simulink model "final_quadruped_180622_veldelay"  (R2021a)
settings: Solver=ode15s  StartTime=0.0  StopTime=2  FixedStep=1e-3  RelTol=1e-5  EnableMultiTasking=on
values from neighbouring files (symbols this model uses):
  foot_x = 8    [bipedparameters.m]    (also in fcn.m; finalrobotParameters.m; finalrobotParameters_110522.m; finalrobotParameters_140522.m)
  foot_y = 6    [bipedparameters.m]    (also in fcn.m; finalrobotParameters.m; finalrobotParameters_110522.m; finalrobotParameters_140522.m)
  foot_z = 1    [bipedparameters.m]    (also in fcn.m; finalrobotParameters.m; finalrobotParameters_110522.m; finalrobotParameters_140522.m)
  height_plane = 0.025    [bipedparameters.m]    (also in finalrobotParameters.m; finalrobotParameters_110522.m; finalrobotParameters_140522.m; finalrobotParameters_240522.m)
  kd_ankle = 1000    [bipedparameters.m]    (also in finalrobotParameters_240522.m)
  kd_hip = 1000    [bipedparameters.m]    (also in finalrobotParameters_240522.m)
  kd_knee = 1000    [bipedparameters.m]    (also in finalrobotParameters_240522.m)
  ki_ankle = 1000    [bipedparameters.m]    (also in finalrobotParameters_240522.m)
  ki_hip = 1000    [bipedparameters.m]    (also in finalrobotParameters_240522.m)
  ki_knee = 2000    [bipedparameters.m]    (also in finalrobotParameters_240522.m)
  kp_ankle = 1000    [bipedparameters.m]    (also in finalrobotParameters_240522.m)
  kp_hip = 1000    [bipedparameters.m]    (also in finalrobotParameters_240522.m)
  kp_knee = 2000    [bipedparameters.m]    (also in finalrobotParameters_240522.m)
  lower_leg_length = 10    [bipedparameters.m]    (also in fcn.m; finalrobotParameters.m; finalrobotParameters_110522.m; finalrobotParameters_140522.m)
  m_ll = density*leg_radius*leg_radius*lower_leg_length*3.141592653589*0.01*0.01*0.01    (= 0.0176714586764)    [bipedparameters.m]    (also in fcn.m; finalrobotParameters_140522.m; finalrobotParameters_240522.m; hdotlb.m)
  m_ul = density*leg_radius*leg_radius*upper_leg_length*3.141592653589*0.01*0.01*0.01    (= 0.0176714586764)    [bipedparameters.m]    (also in fcn.m; finalrobotParameters_140522.m; finalrobotParameters_240522.m; hdotlb.m)
  plane_x = 25    [bipedparameters.m]    (also in finalrobotParameters.m; finalrobotParameters_110522.m; finalrobotParameters_140522.m; finalrobotParameters_240522.m)
  plane_y = 3    [bipedparameters.m]    (also in finalrobotParameters.m; finalrobotParameters_110522.m; finalrobotParameters_140522.m; finalrobotParameters_240522.m)
  torso_offset_x = -0.5    [bipedparameters.m]    (also in finalrobotParameters.m = 10; finalrobotParameters_110522.m = 10; finalrobotParameters_140522.m = 10; finalrobotParameters_240522.m = 10)
  torso_offset_z = -2    [bipedparameters.m]    (also in finalrobotParameters.m; finalrobotParameters_110522.m; finalrobotParameters_140522.m; finalrobotParameters_240522.m)
  torso_x = 5    [bipedparameters.m]    (also in fcn.m = 25; finalrobotParameters.m = 25; finalrobotParameters_110522.m = 25; finalrobotParameters_140522.m = 25)
  torso_y = 10    [bipedparameters.m]    (also in fcn.m = 16; finalrobotParameters.m = 16; finalrobotParameters_110522.m = 16; finalrobotParameters_140522.m = 16)
  torso_z = 8    [bipedparameters.m]    (also in fcn.m = 10; finalrobotParameters.m = 10; finalrobotParameters_110522.m = 10; finalrobotParameters_140522.m = 10)
  upper_leg_length = 10    [bipedparameters.m]    (also in fcn.m; finalrobotParameters.m; finalrobotParameters_110522.m; finalrobotParameters_140522.m)
undefined symbols (not defined in the file or in its folder): sigbuilder_block, X, Y, Z
libraries: nesl_utility x188, sm_lib x71, Contact_Forces_Lib x16, pid_lib x12, fl_lib x3
(part 2 of 8)

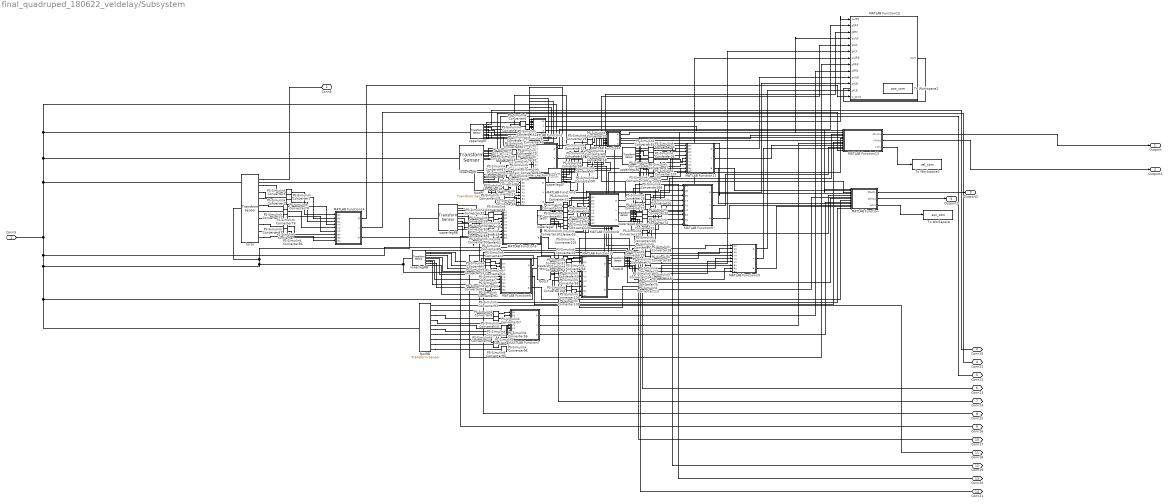
== system final_quadruped_180622_veldelay/Subsystem ==
  MATLAB Function : MATLAB Function  TreatAsAtomicUnit=on
  MATLAB Function1 : MATLAB Function  TreatAsAtomicUnit=on
  MATLAB Function10 : MATLAB Function  TreatAsAtomicUnit=on
  MATLAB Function11 : MATLAB Function  TreatAsAtomicUnit=on
  MATLAB Function12 : MATLAB Function  TreatAsAtomicUnit=on
  MATLAB Function13 : MATLAB Function  TreatAsAtomicUnit=on
  MATLAB Function14 : MATLAB Function  TreatAsAtomicUnit=on
  MATLAB Function15 : MATLAB Function  TreatAsAtomicUnit=on
  MATLAB Function2 : MATLAB Function  TreatAsAtomicUnit=on
  MATLAB Function3 : MATLAB Function  TreatAsAtomicUnit=on
  MATLAB Function4 : MATLAB Function  TreatAsAtomicUnit=on
  MATLAB Function5 : MATLAB Function  TreatAsAtomicUnit=on
  MATLAB Function6 : MATLAB Function  TreatAsAtomicUnit=on
  MATLAB Function7 : MATLAB Function  TreatAsAtomicUnit=on
  MATLAB Function8 : MATLAB Function  TreatAsAtomicUnit=on
  MATLAB Function9 : MATLAB Function  TreatAsAtomicUnit=on
  PS-Simulink Converter{,1..114} (115 alike) : nesl_utility/PS-Simulink Converter  PhysicalDomain=network_engine_domain  SubClassName=ps_output  LeftPortType=input  RightPortType=output  PseudoPeriodic=off  Frequencies=[]  Unit=inherit  AffineConversion=off
      settings: SourceProductBaseCode=PW,SS
  To Workspace : ToWorkspace  VariableName=acc_com  SaveFormat=Timeseries  SampleTime=-1
  To Workspace1 : ToWorkspace  VariableName=vel_com  SaveFormat=Timeseries  SampleTime=-1
  To Workspace2 : ToWorkspace  VariableName=pos_com  SaveFormat=Timeseries  SampleTime=-1
  footLB : sm_lib/Frames and Transforms/Transform Sensor  MeasurementFrame=World  SenseAngle=off  SenseAxis=off  SenseAngle1=off  SenseAngle2=off  SenseAngle3=off  SenseQ=off  SenseR=off  SenseOmegaX=off  SenseOmegaY=off  SenseOmegaZ=off  SenseOmega1=off  SenseOmega2=off  SenseOmega3=off  SenseQDot=off  SenseRDot=off  SenseAlphaX=off  SenseAlphaY=off  SenseAlphaZ=off  SenseAlpha1=off  SenseAlpha2=off  SenseAlpha3=off  SenseQDDot=off  SenseRDDot=off  SenseX=on  SenseY=on  SenseZ=on  SenseRad=off  SenseAzim=off  SenseDist=off  SenseInc=off  SenseXDot=on  SenseYDot=on  SenseZDot=on  SenseRadDot=off  SenseAzimDot=off  SenseDistDot=off  SenseIncDot=off  SenseXDDot=on  SenseYDDot=on  SenseZDDot=on  SenseRadDDot=off  SenseAzimDDot=off  SenseDistDDot=off  SenseIncDDot=off
  footLF : sm_lib/Frames and Transforms/Transform Sensor  MeasurementFrame=World  SenseAngle=off  SenseAxis=off  SenseAngle1=off  SenseAngle2=off  SenseAngle3=off  SenseQ=off  SenseR=off  SenseOmegaX=off  SenseOmegaY=off  SenseOmegaZ=off  SenseOmega1=off  SenseOmega2=off  SenseOmega3=off  SenseQDot=off  SenseRDot=off  SenseAlphaX=off  SenseAlphaY=off  SenseAlphaZ=off  SenseAlpha1=off  SenseAlpha2=off  SenseAlpha3=off  SenseQDDot=off  SenseRDDot=off  SenseX=on  SenseY=on  SenseZ=on  SenseRad=off  SenseAzim=off  SenseDist=off  SenseInc=off  SenseXDot=on  SenseYDot=on  SenseZDot=on  SenseRadDot=off  SenseAzimDot=off  SenseDistDot=off  SenseIncDot=off  SenseXDDot=on  SenseYDDot=on  SenseZDDot=on  SenseRadDDot=off  SenseAzimDDot=off  SenseDistDDot=off  SenseIncDDot=off
  footRB : sm_lib/Frames and Transforms/Transform Sensor  MeasurementFrame=World  SenseAngle=off  SenseAxis=off  SenseAngle1=off  SenseAngle2=off  SenseAngle3=off  SenseQ=off  SenseR=off  SenseOmegaX=off  SenseOmegaY=off  SenseOmegaZ=off  SenseOmega1=off  SenseOmega2=off  SenseOmega3=off  SenseQDot=off  SenseRDot=off  SenseAlphaX=off  SenseAlphaY=off  SenseAlphaZ=off  SenseAlpha1=off  SenseAlpha2=off  SenseAlpha3=off  SenseQDDot=off  SenseRDDot=off  SenseX=on  SenseY=on  SenseZ=on  SenseRad=off  SenseAzim=off  SenseDist=off  SenseInc=off  SenseXDot=on  SenseYDot=on  SenseZDot=on  SenseRadDot=off  SenseAzimDot=off  SenseDistDot=off  SenseIncDot=off  SenseXDDot=on  SenseYDDot=on  SenseZDDot=on  SenseRadDDot=off  SenseAzimDDot=off  SenseDistDDot=off  SenseIncDDot=off
  footRF : sm_lib/Frames and Transforms/Transform Sensor  MeasurementFrame=World  SenseAngle=off  SenseAxis=off  SenseAngle1=off  SenseAngle2=off  SenseAngle3=off  SenseQ=off  SenseR=off  SenseOmegaX=off  SenseOmegaY=off  SenseOmegaZ=off  SenseOmega1=off  SenseOmega2=off  SenseOmega3=off  SenseQDot=off  SenseRDot=off  SenseAlphaX=off  SenseAlphaY=off  SenseAlphaZ=off  SenseAlpha1=off  SenseAlpha2=off  SenseAlpha3=off  SenseQDDot=off  SenseRDDot=off  SenseX=on  SenseY=on  SenseZ=on  SenseRad=off  SenseAzim=off  SenseDist=off  SenseInc=off  SenseXDot=on  SenseYDot=on  SenseZDot=on  SenseRadDot=off  SenseAzimDot=off  SenseDistDot=off  SenseIncDot=off  SenseXDDot=on  SenseYDDot=on  SenseZDDot=on  SenseRadDDot=off  SenseAzimDDot=off  SenseDistDDot=off  SenseIncDDot=off
  lowerlegLB : sm_lib/Frames and Transforms/Transform Sensor  MeasurementFrame=World  SenseAngle=off  SenseAxis=off  SenseAngle1=off  SenseAngle2=off  SenseAngle3=off  SenseQ=off  SenseR=off  SenseOmegaX=off  SenseOmegaY=off  SenseOmegaZ=off  SenseOmega1=off  SenseOmega2=off  SenseOmega3=off  SenseQDot=off  SenseRDot=off  SenseAlphaX=off  SenseAlphaY=off  SenseAlphaZ=off  SenseAlpha1=off  SenseAlpha2=off  SenseAlpha3=off  SenseQDDot=off  SenseRDDot=off  SenseX=on  SenseY=on  SenseZ=on  SenseRad=off  SenseAzim=off  SenseDist=off  SenseInc=off  SenseXDot=on  SenseYDot=on  SenseZDot=on  SenseRadDot=off  SenseAzimDot=off  SenseDistDot=off  SenseIncDot=off  SenseXDDot=on  SenseYDDot=on  SenseZDDot=on  SenseRadDDot=off  SenseAzimDDot=off  SenseDistDDot=off  SenseIncDDot=off
  lowerlegLF : sm_lib/Frames and Transforms/Transform Sensor  MeasurementFrame=World  SenseAngle=off  SenseAxis=off  SenseAngle1=off  SenseAngle2=off  SenseAngle3=off  SenseQ=off  SenseR=off  SenseOmegaX=off  SenseOmegaY=off  SenseOmegaZ=off  SenseOmega1=off  SenseOmega2=off  SenseOmega3=off  SenseQDot=off  SenseRDot=off  SenseAlphaX=off  SenseAlphaY=off  SenseAlphaZ=off  SenseAlpha1=off  SenseAlpha2=off  SenseAlpha3=off  SenseQDDot=off  SenseRDDot=off  SenseX=on  SenseY=on  SenseZ=on  SenseRad=off  SenseAzim=off  SenseDist=off  SenseInc=off  SenseXDot=on  SenseYDot=on  SenseZDot=on  SenseRadDot=off  SenseAzimDot=off  SenseDistDot=off  SenseIncDot=off  SenseXDDot=on  SenseYDDot=on  SenseZDDot=on  SenseRadDDot=off  SenseAzimDDot=off  SenseDistDDot=off  SenseIncDDot=off
  lowerlegRB : sm_lib/Frames and Transforms/Transform Sensor  MeasurementFrame=World  SenseAngle=off  SenseAxis=off  SenseAngle1=off  SenseAngle2=off  SenseAngle3=off  SenseQ=off  SenseR=off  SenseOmegaX=off  SenseOmegaY=off  SenseOmegaZ=off  SenseOmega1=off  SenseOmega2=off  SenseOmega3=off  SenseQDot=off  SenseRDot=off  SenseAlphaX=off  SenseAlphaY=off  SenseAlphaZ=off  SenseAlpha1=off  SenseAlpha2=off  SenseAlpha3=off  SenseQDDot=off  SenseRDDot=off  SenseX=on  SenseY=on  SenseZ=on  SenseRad=off  SenseAzim=off  SenseDist=off  SenseInc=off  SenseXDot=on  SenseYDot=on  SenseZDot=on  SenseRadDot=off  SenseAzimDot=off  SenseDistDot=off  SenseIncDot=off  SenseXDDot=on  SenseYDDot=on  SenseZDDot=on  SenseRadDDot=off  SenseAzimDDot=off  SenseDistDDot=off  SenseIncDDot=off
  lowerlegRF : sm_lib/Frames and Transforms/Transform Sensor  MeasurementFrame=World  SenseAngle=off  SenseAxis=off  SenseAngle1=off  SenseAngle2=off  SenseAngle3=off  SenseQ=off  SenseR=off  SenseOmegaX=off  SenseOmegaY=off  SenseOmegaZ=off  SenseOmega1=off  SenseOmega2=off  SenseOmega3=off  SenseQDot=off  SenseRDot=off  SenseAlphaX=off  SenseAlphaY=off  SenseAlphaZ=off  SenseAlpha1=off  SenseAlpha2=off  SenseAlpha3=off  SenseQDDot=off  SenseRDDot=off  SenseX=on  SenseY=on  SenseZ=on  SenseRad=off  SenseAzim=off  SenseDist=off  SenseInc=off  SenseXDot=on  SenseYDot=on  SenseZDot=on  SenseRadDot=off  SenseAzimDot=off  SenseDistDot=off  SenseIncDot=off  SenseXDDot=on  SenseYDDot=on  SenseZDDot=on  SenseRadDDot=off  SenseAzimDDot=off  SenseDistDDot=off  SenseIncDDot=off
  torso : sm_lib/Frames and Transforms/Transform Sensor  MeasurementFrame=World  SenseAngle=off  SenseAxis=off  SenseAngle1=off  SenseAngle2=off  SenseAngle3=off  SenseQ=off  SenseR=off  SenseOmegaX=off  SenseOmegaY=off  SenseOmegaZ=off  SenseOmega1=off  SenseOmega2=off  SenseOmega3=off  SenseQDot=off  SenseRDot=off  SenseAlphaX=off  SenseAlphaY=off  SenseAlphaZ=off  SenseAlpha1=off  SenseAlpha2=off  SenseAlpha3=off  SenseQDDot=off  SenseRDDot=off  SenseX=on  SenseY=on  SenseZ=on  SenseRad=off  SenseAzim=off  SenseDist=off  SenseInc=off  SenseXDot=on  SenseYDot=on  SenseZDot=on  SenseRadDot=off  SenseAzimDot=off  SenseDistDot=off  SenseIncDot=off  SenseXDDot=on  SenseYDDot=on  SenseZDDot=on  SenseRadDDot=off  SenseAzimDDot=off  SenseDistDDot=off  SenseIncDDot=off
  upperlegLB1 : sm_lib/Frames and Transforms/Transform Sensor  MeasurementFrame=World  SenseAngle=off  SenseAxis=off  SenseAngle1=off  SenseAngle2=off  SenseAngle3=off  SenseQ=off  SenseR=off  SenseOmegaX=off  SenseOmegaY=off  SenseOmegaZ=off  SenseOmega1=off  SenseOmega2=off  SenseOmega3=off  SenseQDot=off  SenseRDot=off  SenseAlphaX=off  SenseAlphaY=off  SenseAlphaZ=off  SenseAlpha1=off  SenseAlpha2=off  SenseAlpha3=off  SenseQDDot=off  SenseRDDot=off  SenseX=on  SenseY=on  SenseZ=on  SenseRad=off  SenseAzim=off  SenseDist=off  SenseInc=off  SenseXDot=on  SenseYDot=on  SenseZDot=on  SenseRadDot=off  SenseAzimDot=off  SenseDistDot=off  SenseIncDot=off  SenseXDDot=on  SenseYDDot=on  SenseZDDot=on  SenseRadDDot=off  SenseAzimDDot=off  SenseDistDDot=off  SenseIncDDot=off
  upperlegLF : sm_lib/Frames and Transforms/Transform Sensor  MeasurementFrame=World  SenseAngle=off  SenseAxis=off  SenseAngle1=off  SenseAngle2=off  SenseAngle3=off  SenseQ=off  SenseR=off  SenseOmegaX=off  SenseOmegaY=off  SenseOmegaZ=off  SenseOmega1=off  SenseOmega2=off  SenseOmega3=off  SenseQDot=off  SenseRDot=off  SenseAlphaX=off  SenseAlphaY=off  SenseAlphaZ=off  SenseAlpha1=off  SenseAlpha2=off  SenseAlpha3=off  SenseQDDot=off  SenseRDDot=off  SenseX=on  SenseY=on  SenseZ=on  SenseRad=off  SenseAzim=off  SenseDist=off  SenseInc=off  SenseXDot=on  SenseYDot=on  SenseZDot=on  SenseRadDot=off  SenseAzimDot=off  SenseDistDot=off  SenseIncDot=off  SenseXDDot=on  SenseYDDot=on  SenseZDDot=on  SenseRadDDot=off  SenseAzimDDot=off  SenseDistDDot=off  SenseIncDDot=off
  upperlegRB : sm_lib/Frames and Transforms/Transform Sensor  MeasurementFrame=World  SenseAngle=off  SenseAxis=off  SenseAngle1=off  SenseAngle2=off  SenseAngle3=off  SenseQ=off  SenseR=off  SenseOmegaX=off  SenseOmegaY=off  SenseOmegaZ=off  SenseOmega1=off  SenseOmega2=off  SenseOmega3=off  SenseQDot=off  SenseRDot=off  SenseAlphaX=off  SenseAlphaY=off  SenseAlphaZ=off  SenseAlpha1=off  SenseAlpha2=off  SenseAlpha3=off  SenseQDDot=off  SenseRDDot=off  SenseX=on  SenseY=on  SenseZ=on  SenseRad=off  SenseAzim=off  SenseDist=off  SenseInc=off  SenseXDot=on  SenseYDot=on  SenseZDot=on  SenseRadDot=off  SenseAzimDot=off  SenseDistDot=off  SenseIncDot=off  SenseXDDot=on  SenseYDDot=on  SenseZDDot=on  SenseRadDDot=off  SenseAzimDDot=off  SenseDistDDot=off  SenseIncDDot=off
  upperlegRF : sm_lib/Frames and Transforms/Transform Sensor  MeasurementFrame=World  SenseAngle=off  SenseAxis=off  SenseAngle1=off  SenseAngle2=off  SenseAngle3=off  SenseQ=off  SenseR=off  SenseOmegaX=off  SenseOmegaY=off  SenseOmegaZ=off  SenseOmega1=off  SenseOmega2=off  SenseOmega3=off  SenseQDot=off  SenseRDot=off  SenseAlphaX=off  SenseAlphaY=off  SenseAlphaZ=off  SenseAlpha1=off  SenseAlpha2=off  SenseAlpha3=off  SenseQDDot=off  SenseRDDot=off  SenseX=on  SenseY=on  SenseZ=on  SenseRad=off  SenseAzim=off  SenseDist=off  SenseInc=off  SenseXDot=on  SenseYDot=on  SenseZDot=on  SenseRadDot=off  SenseAzimDot=off  SenseDistDot=off  SenseIncDot=off  SenseXDDot=on  SenseYDDot=on  SenseZDDot=on  SenseRadDDot=off  SenseAzimDDot=off  SenseDistDDot=off  SenseIncDDot=off
  Conn5 : PMIOPort  Side=Left
  Conn4 : PMIOPort  Port=2  Side=Right
  Conn10 : PMIOPort  Port=3  Side=Right
  Conn11 : PMIOPort  Port=4  Side=Right
  Conn12 : PMIOPort  Port=5  Side=Right
  Conn13 : PMIOPort  Port=6  Side=Right
  Conn14 : PMIOPort  Port=7  Side=Right
  Conn15 : PMIOPort  Port=8  Side=Right
  Conn16 : PMIOPort  Port=9  Side=Right
  Conn17 : PMIOPort  Port=10  Side=Right
  Conn18 : PMIOPort  Port=11  Side=Right
  Conn19 : PMIOPort  Port=12  Side=Right
  Conn20 : PMIOPort  Port=13  Side=Right
  Conn21 : PMIOPort  Port=14  Side=Right
  Outport : Outport
  Outport1 : Outport  Port=2
  Outport2 : Outport  Port=3
  Outport3 : Outport  Port=4
  wires:
  PS-Simulink Converter10/1 -> MATLAB Function7/2(py)
  PS-Simulink Converter13/1 -> MATLAB Function2/1(px)
  MATLAB Function12/2(v) -> MATLAB Function13/10(vulLB)
  PS-Simulink Converter36/1 -> MATLAB Function12/3(pz)
  PS-Simulink Converter14/1 -> MATLAB Function2/2(py)
  PS-Simulink Converter9/1 -> MATLAB Function7/1(px)
  PS-Simulink Converter11/1 -> MATLAB Function7/3(pz)
  PS-Simulink Converter8/1 -> MATLAB Function1/2(py)
  PS-Simulink Converter7/1 -> MATLAB Function6/3(pz)
  PS-Simulink Converter38/1 -> MATLAB Function5/2(py)
  PS-Simulink Converter16/1 -> MATLAB Function3/4(vx)
  MATLAB Function9/2(v) -> MATLAB Function13/11(vllLB)
  MATLAB Function1/2(v) -> MATLAB Function13/1(vulRF)
  PS-Simulink Converter17/1 -> MATLAB Function3/5(vy)
  PS-Simulink Converter28/1 -> MATLAB Function10/1(px)
  PS-Simulink Converter21/1 -> MATLAB Function4/3(pz)
  PS-Simulink Converter18/1 -> MATLAB Function3/6(vz)
  PS-Simulink Converter6/1 -> MATLAB Function1/1(px)
  PS-Simulink Converter19/1 -> MATLAB Function4/1(px)
  PS-Simulink Converter5/1 -> MATLAB Function6/2(py)
  PS-Simulink Converter20/1 -> MATLAB Function4/2(py)
  PS-Simulink Converter12/1 -> MATLAB Function1/3(pz)
  PS-Simulink Converter15/1 -> MATLAB Function2/3(pz)
  PS-Simulink Converter39/1 -> MATLAB Function5/3(pz)
  MATLAB Function2/2(v) -> MATLAB Function13/2(vllRF)
  MATLAB Function10/2(v) -> MATLAB Function13/12(vfLB)
  PS-Simulink Converter27/1 -> MATLAB Function9/3(pz)
  PS-Simulink Converter4/1 -> MATLAB Function6/1(px)
  PS-Simulink Converter25/1 -> MATLAB Function9/1(px)
  PS-Simulink Converter37/1 -> MATLAB Function5/1(px)
  PS-Simulink Converter26/1 -> MATLAB Function9/2(py)
  PS-Simulink Converter24/1 -> MATLAB Function8/3(pz)
  PS-Simulink Converter22/1 -> MATLAB Function8/1(px)
  PS-Simulink Converter23/1 -> MATLAB Function8/2(py)
  PS-Simulink Converter34/1 -> MATLAB Function12/1(px)
  PS-Simulink Converter35/1 -> MATLAB Function12/2(py)
  MATLAB Function7/2(v) -> MATLAB Function13/9(vfRB)
  MATLAB Function6/2(v) -> MATLAB Function13/8(vllRB)
  MATLAB Function5/2(v) -> MATLAB Function13/7(vulRB)
  MATLAB Function11/2(v) -> MATLAB Function13/6(vfLF)
  PS-Simulink Converter33/1 -> MATLAB Function11/3(pz)
  MATLAB Function8/2(v) -> MATLAB Function13/5(vllLF)
  MATLAB Function4/2(v) -> MATLAB Function13/4(vulLF)
  MATLAB Function3/2(v) -> MATLAB Function13/3(vfRF)
  PS-Simulink Converter32/1 -> MATLAB Function11/2(py)
  PS-Simulink Converter31/1 -> MATLAB Function11/1(px)
  PS-Simulink Converter30/1 -> MATLAB Function10/3(pz)
  PS-Simulink Converter29/1 -> MATLAB Function10/2(py)
  PS-Simulink Converter3/1 -> MATLAB Function14/1(px)
  PS-Simulink Converter1/1 -> MATLAB Function14/2(py)
  PS-Simulink Converter2/1 -> MATLAB Function14/3(pz)
  MATLAB Function14/2(v) -> MATLAB Function13/13(v_torso)
  MATLAB Function13/1(Mvcm) -> Outport/1
  MATLAB Function13/2(vlinks) -> Outport1/1
  PS-Simulink Converter40/1 -> MATLAB Function1/4(vx)
  PS-Simulink Converter41/1 -> MATLAB Function1/5(vy)
  PS-Simulink Converter42/1 -> MATLAB Function1/6(vz)
  PS-Simulink Converter43/1 -> MATLAB Function2/4(vx)
  PS-Simulink Converter44/1 -> MATLAB Function2/5(vy)
  PS-Simulink Converter45/1 -> MATLAB Function2/6(vz)
  PS-Simulink Converter46/1 -> MATLAB Function3/7(ax)
  PS-Simulink Converter47/1 -> MATLAB Function3/8(ay)
  PS-Simulink Converter48/1 -> MATLAB Function3/9(az)
  PS-Simulink Converter49/1 -> MATLAB Function5/4(vx)
  PS-Simulink Converter50/1 -> MATLAB Function5/5(vy)
  PS-Simulink Converter51/1 -> MATLAB Function5/6(vz)
  PS-Simulink Converter52/1 -> MATLAB Function6/4(vx)
  PS-Simulink Converter53/1 -> MATLAB Function6/5(vy)
  PS-Simulink Converter54/1 -> MATLAB Function6/6(vz)
  PS-Simulink Converter55/1 -> MATLAB Function7/5(vy)
  PS-Simulink Converter57/1 -> MATLAB Function7/4(vx)
  PS-Simulink Converter56/1 -> MATLAB Function7/6(vz)
  PS-Simulink Converter58/1 -> MATLAB Function4/4(vx)
  PS-Simulink Converter59/1 -> MATLAB Function4/5(vy)
  PS-Simulink Converter60/1 -> MATLAB Function4/6(vz)
  PS-Simulink Converter61/1 -> MATLAB Function8/4(vx)
  PS-Simulink Converter62/1 -> MATLAB Function8/5(vy)
  PS-Simulink Converter63/1 -> MATLAB Function8/6(vz)
  PS-Simulink Converter64/1 -> MATLAB Function11/4(vx)
  PS-Simulink Converter65/1 -> MATLAB Function11/5(vy)
  PS-Simulink Converter66/1 -> MATLAB Function11/6(vz)
  PS-Simulink Converter67/1 -> MATLAB Function12/4(vx)
  PS-Simulink Converter68/1 -> MATLAB Function12/5(vy)
  PS-Simulink Converter69/1 -> MATLAB Function12/6(vz)
  PS-Simulink Converter70/1 -> MATLAB Function9/4(vx)
  PS-Simulink Converter71/1 -> MATLAB Function9/5(vy)
  PS-Simulink Converter72/1 -> MATLAB Function9/6(vz)
  PS-Simulink Converter73/1 -> MATLAB Function10/4(vx)
  PS-Simulink Converter74/1 -> MATLAB Function10/5(vy)
  PS-Simulink Converter75/1 -> MATLAB Function10/6(vz)
  PS-Simulink Converter78/1 -> MATLAB Function14/4(vx)
  PS-Simulink Converter76/1 -> MATLAB Function14/5(vy)
  PS-Simulink Converter77/1 -> MATLAB Function14/6(vz)
  MATLAB Function14/3(a) -> MATLAB Function/13(a_torso)
  MATLAB Function1/3(a) -> MATLAB Function/1(aulRF)
  MATLAB Function2/3(a) -> MATLAB Function/2(allRF)
  MATLAB Function3/3(a) -> MATLAB Function/3(afRF)
  MATLAB Function4/3(a) -> MATLAB Function/4(aulLF)
  MATLAB Function8/3(a) -> MATLAB Function/5(allLF)
  MATLAB Function11/3(a) -> MATLAB Function/6(afLF)
  MATLAB Function5/3(a) -> MATLAB Function/7(aulRB)
  MATLAB Function6/3(a) -> MATLAB Function/8(allRB)
  MATLAB Function7/3(a) -> MATLAB Function/9(afRB)
  MATLAB Function12/3(a) -> MATLAB Function/10(aulLB)
  MATLAB Function9/3(a) -> MATLAB Function/11(allLB)
  MATLAB Function10/3(a) -> MATLAB Function/12(afLB)
  MATLAB Function/1(Macm) -> Outport2/1
  MATLAB Function/2(alinks) -> Outport3/1
  MATLAB Function/3(acm) -> To Workspace/1
  MATLAB Function13/3(vcm) -> To Workspace1/1
  PS-Simulink Converter79/1 -> MATLAB Function1/7(ax)
  PS-Simulink Converter80/1 -> MATLAB Function1/8(ay)
  PS-Simulink Converter81/1 -> MATLAB Function1/9(az)
  PS-Simulink Converter82/1 -> MATLAB Function2/7(ax)
  PS-Simulink Converter83/1 -> MATLAB Function3/1(px)
  PS-Simulink Converter84/1 -> MATLAB Function3/2(py)
  PS-Simulink Converter85/1 -> MATLAB Function3/3(pz)
  PS-Simulink Converter/1 -> MATLAB Function14/7(ax)
  PS-Simulink Converter87/1 -> MATLAB Function14/8(ay)
  PS-Simulink Converter86/1 -> MATLAB Function14/9(az)
  PS-Simulink Converter88/1 -> MATLAB Function5/7(ax)
  PS-Simulink Converter89/1 -> MATLAB Function5/8(ay)
  PS-Simulink Converter90/1 -> MATLAB Function5/9(az)
  PS-Simulink Converter91/1 -> MATLAB Function6/7(ax)
  PS-Simulink Converter92/1 -> MATLAB Function6/8(ay)
  PS-Simulink Converter93/1 -> MATLAB Function6/9(az)
  PS-Simulink Converter94/1 -> MATLAB Function7/7(ax)
  PS-Simulink Converter95/1 -> MATLAB Function7/8(ay)
  PS-Simulink Converter96/1 -> MATLAB Function7/9(az)
  PS-Simulink Converter97/1 -> MATLAB Function4/7(ax)
  PS-Simulink Converter98/1 -> MATLAB Function4/8(ay)
  PS-Simulink Converter99/1 -> MATLAB Function4/9(az)
  PS-Simulink Converter100/1 -> MATLAB Function8/7(ax)
  PS-Simulink Converter101/1 -> MATLAB Function8/8(ay)
  PS-Simulink Converter102/1 -> MATLAB Function8/9(az)
  PS-Simulink Converter103/1 -> MATLAB Function11/7(ax)
  PS-Simulink Converter104/1 -> MATLAB Function11/8(ay)
  PS-Simulink Converter105/1 -> MATLAB Function11/9(az)
  PS-Simulink Converter107/1 -> MATLAB Function12/7(ax)
  PS-Simulink Converter108/1 -> MATLAB Function12/8(ay)
  PS-Simulink Converter109/1 -> MATLAB Function12/9(az)
  PS-Simulink Converter106/1 -> MATLAB Function9/7(ax)
  PS-Simulink Converter110/1 -> MATLAB Function9/8(ay)
  PS-Simulink Converter111/1 -> MATLAB Function9/9(az)
  PS-Simulink Converter112/1 -> MATLAB Function10/7(ax)
  PS-Simulink Converter113/1 -> MATLAB Function10/8(ay)
  PS-Simulink Converter114/1 -> MATLAB Function10/9(az)
  MATLAB Function1/1(p) -> MATLAB Function15/1(pulRF)
  MATLAB Function2/1(p) -> MATLAB Function15/2(pllRF)
  MATLAB Function3/1(p) -> MATLAB Function15/3(pfRF)
  MATLAB Function4/1(p) -> MATLAB Function15/4(pulLF)
  MATLAB Function8/1(p) -> MATLAB Function15/5(pllLF)
  MATLAB Function11/1(p) -> MATLAB Function15/6(pfLF)
  MATLAB Function5/1(p) -> MATLAB Function15/7(pulRB)
  MATLAB Function6/1(p) -> MATLAB Function15/8(pllRB)
  MATLAB Function7/1(p) -> MATLAB Function15/9(pfRB)
  MATLAB Function12/1(p) -> MATLAB Function15/10(pulLB)
  MATLAB Function9/1(p) -> MATLAB Function15/11(pllLB)
  MATLAB Function10/1(p) -> MATLAB Function15/12(pfLB)
  MATLAB Function14/1(p) -> MATLAB Function15/13(p_torso)
  MATLAB Function15/1(pcm) -> To Workspace2/1
  connections:
  footRB/RConn4 -- PS-Simulink Converter11/LConn1
  lowerlegLF/RConn2 -- PS-Simulink Converter22/LConn1
  upperlegLF/RConn4 -- PS-Simulink Converter21/LConn1
  footLB/RConn2 -- PS-Simulink Converter28/LConn1
  upperlegLB1/RConn1 -- Conn19/RConn1
  footLF/RConn2 -- PS-Simulink Converter31/LConn1
  lowerlegLB/LConn1 -- footLB/LConn1 -- torso/LConn1 -- upperlegRB/LConn1 -- footRB/LConn1 -- footLF/LConn1 -- upperlegLF/LConn1 -- upperlegRF/LConn1 -- lowerlegRF/LConn1 -- footRF/LConn1 -- Conn5/RConn1 -- lowerlegLF/LConn1 -- lowerlegRB/LConn1 -- upperlegLB1/LConn1
  lowerlegRB/RConn4 -- PS-Simulink Converter7/LConn1
  Conn17/RConn1 -- lowerlegRB/RConn1
  upperlegLF/RConn2 -- PS-Simulink Converter19/LConn1
  upperlegLF/RConn3 -- PS-Simulink Converter20/LConn1
  lowerlegRF/RConn3 -- PS-Simulink Converter14/LConn1
  footLB/RConn4 -- PS-Simulink Converter30/LConn1
  footRB/RConn3 -- PS-Simulink Converter10/LConn1
  upperlegRB/RConn3 -- PS-Simulink Converter38/LConn1
  lowerlegRF/RConn2 -- PS-Simulink Converter13/LConn1
  upperlegRB/RConn4 -- PS-Simulink Converter39/LConn1
  upperlegRB/RConn2 -- PS-Simulink Converter37/LConn1
  upperlegRF/RConn2 -- PS-Simulink Converter6/LConn1
  footLB/RConn1 -- Conn21/RConn1
  lowerlegRF/RConn4 -- PS-Simulink Converter15/LConn1
  lowerlegLF/RConn4 -- PS-Simulink Converter24/LConn1
  upperlegLB1/RConn4 -- PS-Simulink Converter36/LConn1
  footRB/RConn2 -- PS-Simulink Converter9/LConn1
  upperlegRF/RConn4 -- PS-Simulink Converter12/LConn1
  upperlegRF/RConn3 -- PS-Simulink Converter8/LConn1
  lowerlegLF/RConn3 -- PS-Simulink Converter23/LConn1
  lowerlegRB/RConn3 -- PS-Simulink Converter5/LConn1
  lowerlegRB/RConn2 -- PS-Simulink Converter4/LConn1
  lowerlegLB/RConn3 -- PS-Simulink Converter26/LConn1
  lowerlegLB/RConn4 -- PS-Simulink Converter27/LConn1
  lowerlegLB/RConn2 -- PS-Simulink Converter25/LConn1
  lowerlegLB/RConn1 -- Conn20/RConn1
  upperlegLB1/RConn3 -- PS-Simulink Converter35/LConn1
  upperlegLB1/RConn2 -- PS-Simulink Converter34/LConn1
  upperlegRF/RConn1 -- Conn10/RConn1
  upperlegLF/RConn1 -- Conn13/RConn1
  footLF/RConn3 -- PS-Simulink Converter32/LConn1
  footLF/RConn4 -- PS-Simulink Converter33/LConn1
  footLB/RConn3 -- PS-Simulink Converter29/LConn1
  Conn18/RConn1 -- footRB/RConn1
  footLF/RConn1 -- Conn15/RConn1
  Conn16/RConn1 -- upperlegRB/RConn1
  lowerlegLF/RConn1 -- Conn14/RConn1
  Conn11/RConn1 -- lowerlegRF/RConn1
  footRF/RConn1 -- Conn12/RConn1
  torso/RConn1 -- Conn4/RConn1
  torso/RConn3 -- PS-Simulink Converter1/LConn1
  torso/RConn2 -- PS-Simulink Converter3/LConn1
  torso/RConn4 -- PS-Simulink Converter2/LConn1
  upperlegRF/RConn5 -- PS-Simulink Converter40/LConn1
  upperlegRF/RConn6 -- PS-Simulink Converter41/LConn1
  upperlegRF/RConn7 -- PS-Simulink Converter42/LConn1
  lowerlegRF/RConn5 -- PS-Simulink Converter43/LConn1
  lowerlegRF/RConn6 -- PS-Simulink Converter44/LConn1
  lowerlegRF/RConn7 -- PS-Simulink Converter45/LConn1
  upperlegRB/RConn5 -- PS-Simulink Converter49/LConn1
  upperlegRB/RConn6 -- PS-Simulink Converter50/LConn1
  upperlegRB/RConn7 -- PS-Simulink Converter51/LConn1
  PS-Simulink Converter52/LConn1 -- lowerlegRB/RConn5
  PS-Simulink Converter53/LConn1 -- lowerlegRB/RConn6
  PS-Simulink Converter54/LConn1 -- lowerlegRB/RConn7
  footRB/RConn5 -- PS-Simulink Converter57/LConn1
  footRB/RConn6 -- PS-Simulink Converter55/LConn1
  footRB/RConn7 -- PS-Simulink Converter56/LConn1
  upperlegLF/RConn5 -- PS-Simulink Converter58/LConn1
  upperlegLF/RConn6 -- PS-Simulink Converter59/LConn1
  upperlegLF/RConn7 -- PS-Simulink Converter60/LConn1
  lowerlegLF/RConn5 -- PS-Simulink Converter61/LConn1
  lowerlegLF/RConn6 -- PS-Simulink Converter62/LConn1
  lowerlegLF/RConn7 -- PS-Simulink Converter63/LConn1
  footLF/RConn5 -- PS-Simulink Converter64/LConn1
  footLF/RConn6 -- PS-Simulink Converter65/LConn1
  footLF/RConn7 -- PS-Simulink Converter66/LConn1
  upperlegLB1/RConn5 -- PS-Simulink Converter67/LConn1
  upperlegLB1/RConn6 -- PS-Simulink Converter68/LConn1
  upperlegLB1/RConn7 -- PS-Simulink Converter69/LConn1
  lowerlegLB/RConn5 -- PS-Simulink Converter70/LConn1
  lowerlegLB/RConn6 -- PS-Simulink Converter71/LConn1
  lowerlegLB/RConn7 -- PS-Simulink Converter72/LConn1
  footLB/RConn5 -- PS-Simulink Converter73/LConn1
  footLB/RConn6 -- PS-Simulink Converter74/LConn1
  footLB/RConn7 -- PS-Simulink Converter75/LConn1
  torso/RConn5 -- PS-Simulink Converter78/LConn1
  torso/RConn6 -- PS-Simulink Converter76/LConn1
  torso/RConn7 -- PS-Simulink Converter77/LConn1
  upperlegRF/RConn8 -- PS-Simulink Converter79/LConn1
  upperlegRF/RConn9 -- PS-Simulink Converter80/LConn1
  upperlegRF/RConn10 -- PS-Simulink Converter81/LConn1
  footRF/RConn2 -- PS-Simulink Converter83/LConn1
  footRF/RConn3 -- PS-Simulink Converter84/LConn1
  footRF/RConn4 -- PS-Simulink Converter85/LConn1
  footRF/RConn5 -- PS-Simulink Converter16/LConn1
  footRF/RConn6 -- PS-Simulink Converter17/LConn1
  footRF/RConn7 -- PS-Simulink Converter18/LConn1
  footRF/RConn8 -- PS-Simulink Converter46/LConn1
  footRF/RConn9 -- PS-Simulink Converter47/LConn1
  footRF/RConn10 -- PS-Simulink Converter48/LConn1
  torso/RConn8 -- PS-Simulink Converter/LConn1
  torso/RConn9 -- PS-Simulink Converter87/LConn1
  torso/RConn10 -- PS-Simulink Converter86/LConn1
  upperlegRB/RConn8 -- PS-Simulink Converter88/LConn1
  upperlegRB/RConn9 -- PS-Simulink Converter89/LConn1
  upperlegRB/RConn10 -- PS-Simulink Converter90/LConn1
  lowerlegRB/RConn8 -- PS-Simulink Converter91/LConn1
  lowerlegRB/RConn9 -- PS-Simulink Converter92/LConn1
  PS-Simulink Converter93/LConn1 -- lowerlegRB/RConn10
  footRB/RConn8 -- PS-Simulink Converter94/LConn1
  footRB/RConn9 -- PS-Simulink Converter95/LConn1
  footRB/RConn10 -- PS-Simulink Converter96/LConn1
  upperlegLF/RConn8 -- PS-Simulink Converter97/LConn1
  upperlegLF/RConn9 -- PS-Simulink Converter98/LConn1
  upperlegLF/RConn10 -- PS-Simulink Converter99/LConn1
  lowerlegLF/RConn8 -- PS-Simulink Converter100/LConn1
  lowerlegLF/RConn9 -- PS-Simulink Converter101/LConn1
  lowerlegLF/RConn10 -- PS-Simulink Converter102/LConn1
  footLF/RConn8 -- PS-Simulink Converter103/LConn1
  footLF/RConn9 -- PS-Simulink Converter104/LConn1
  footLF/RConn10 -- PS-Simulink Converter105/LConn1
  upperlegLB1/RConn8 -- PS-Simulink Converter107/LConn1
  upperlegLB1/RConn9 -- PS-Simulink Converter108/LConn1
  upperlegLB1/RConn10 -- PS-Simulink Converter109/LConn1
  lowerlegLB/RConn8 -- PS-Simulink Converter106/LConn1
  lowerlegLB/RConn9 -- PS-Simulink Converter110/LConn1
  lowerlegLB/RConn10 -- PS-Simulink Converter111/LConn1
  footLB/RConn8 -- PS-Simulink Converter112/LConn1
  footLB/RConn9 -- PS-Simulink Converter113/LConn1
  footLB/RConn10 -- PS-Simulink Converter114/LConn1
